simulink model "TrimnLan"  (R2022b)
settings: Solver=VariableStepAuto  StartTime=0.0  StopTime=50  RelTol=1e-3
undefined symbols (not defined in the file or in its folder): A, B, C, D
settings Model: Creator=samue  LastModifiedBy=samue

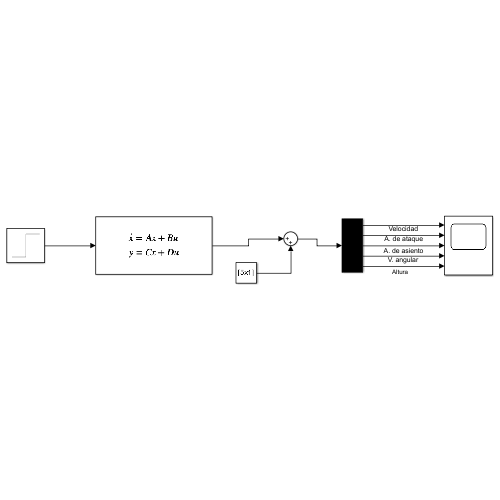
[thumbnail: Simulink's stored preview of the top-level diagram]
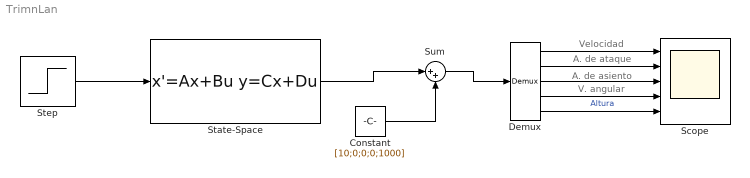
== system TrimnLan ==
  note: V. angular
  note: A. de asiento
  note: A. de ataque
  note: Velocidad
  Constant : Constant  Value=[10;0;0;0;1000]
  Demux : Demux  Outputs=5
  Scope : Scope  NumInputPorts=5
  State-Space : StateSpace  A=A  B=B  C=C  D=D  InitialCondition=[0,0,0,0,0]
  Step : Step  After=[1,0]  SampleTime=0
  Sum : Sum  Inputs=|++
  wires:
  Demux/1 -> Scope/1
  Demux/2 -> Scope/2
  Demux/3 -> Scope/3
  Demux/4 -> Scope/4
  Demux/5 -> Scope/5  "Altura"
  Sum/1 -> Demux/1
  State-Space/1 -> Sum/1
  Constant/1 -> Sum/2
  Step/1 -> State-Space/1
